simulink model "OvercurrentProtection"  (R2024a)
settings: Solver=ode23t  StartTime=0.0  StopTime=simulation.simTime  MaxStep=simulation.maxStepSize  RelTol=1e-3  AbsTol=1e-3
PostLoadFcn:
  | run('OvercurrentProtectionInput.mlx');
  | run('OvercurrentProtectionEstimateSettings.m');
InitFcn:
  | run('OvercurrentProtectionEstimateSettings.m');
undefined symbols (not defined in the file): distributionLine1, distributionLine2, fault, load, protection, relay1, relay2, source
libraries: ee_lib x27, fl_lib x17, eeGeneralControl x8, nesl_utility x7, simulink x4, simulink_extras x4
(part 1 of 2)
CloseFcn:
  | try, close(h1_OvercurrentProtectionPhase), end
  | clear h1_OvercurrentProtectionPhase
  | try, close(h2_OvercurrentProtectionEarth), end
  | clear h2_OvercurrentProtectionEarth
  | clear source;
  | clear transformer;
  | clear distributionLine1;
  | clear distributionLine2;
  | clear load;
  | clear sensor1;
  | clear sensor2;
  | clear fault;
  | clear protection;
  | clear maskParameter;
  | clear simlog_OvercurrentProtection;
  | clear simulation;
  | clear relay1;
  | clear relay2;
  | clear plotVar;
  | clear relayType;
  | clear mask;
Description:
  | Overcurrent Relay Protection in AC Microgrid
settings Model: Creator=The MathWorks, Inc.  LastModifiedBy=The MathWorks, Inc.
settings SolverCC: MaxConsecutiveZCs=100000  MaxConsecutiveMinStep=1000  MaxZcPerStep=1
settings DataIOCC: SaveOutput=off  SignalLogging=off  DSMLogging=off  SaveTime=off  ReturnWorkspaceOutputs=off
settings OptimizationCC: ReuseModelBlockBuffer=off
settings DebuggingCC: UnconnectedInputMsg=warning  UnconnectedOutputMsg=warning  UnconnectedLineMsg=warning
settings ModelReferenceCC: EnableRefExpFcnMdlSchedulingChecks=on
settings RTWCC: GPUComputeCapability=3.5  DLArmComputeVersion=19.05
settings SimscapeCC: SimscapeLogType=all  SimscapeLogName=simlog_OvercurrentProtection  SimscapeLogLimitData=off

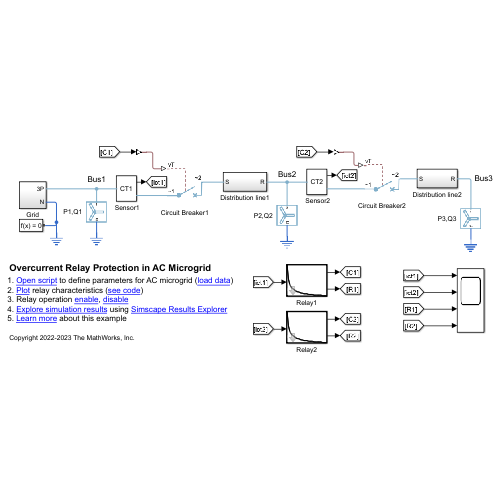
[thumbnail: Simulink's stored preview of the top-level diagram]
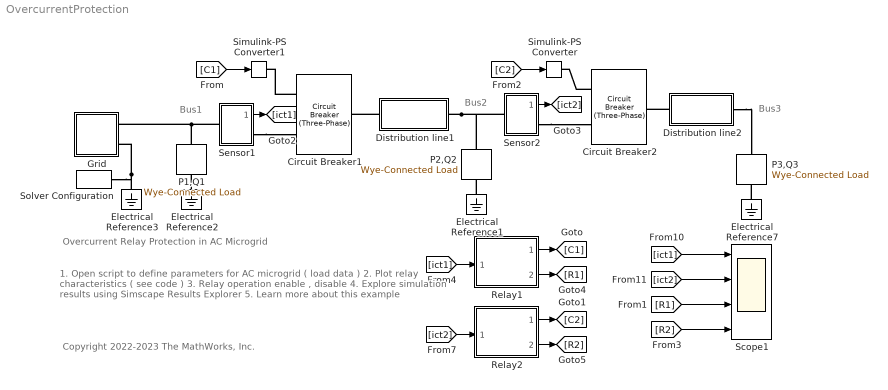
== system OvercurrentProtection ==
  note: Bus1
  note: Bus2
  note: Bus3
  note: Copyright 2022-2023 The MathWorks, Inc.
  note: Overcurrent Relay Protection in AC Microgrid
  note: 1. Open script to define parameters for AC microgrid ( load data )
      | 2. Plot relay characteristics ( see code )
      | 3. Relay operation enable , disable
      | 4. Explore simulation results using Simscape Results Explorer
      | 5. Learn more about this example
  " P2,Q2" : ee_lib/Passive/RLC Assemblies/Wye-Connected Load  parameterization=ee.enum.rlc.parameterization.ratedpower  component_structure=ee.enum.rlc.structure.R  component_structure_PQ=ee.enum.rlc.structure.SeriesRL  R=1 Ohm  L=1e-3 H  C=1e-6 F  VRated=transformer.secVoltage V  FRated=source.ratedFrequency Hz  P=load.P2 W  Qpos=load.Q2 V*A  Qneg=-1e2 V*A  R_parasitic=1e-6 Ohm  G_parasitic=1e-6 1/Ohm  R_parasitic_PQ=1e-6 Ohm  G_parasitic_PQ=1e-6 1/Ohm  Vmag0=33 kV  Vang0=0 deg  Freq0=50 Hz  IL_specify=off  IL_priority=High  IL=[ 0 0 0 ] A  IL_nominal_specify=off  IL_nominal_value=1  IL_nominal_unit=A  VC_specify=off  VC_priority=High  VC=[ 0 0 0 ] V  VC_nominal_specify=off  VC_nominal_value=1  VC_nominal_unit=V
  " Sensor1" : Subsystem
      mask Display: disp('CT1')
  " Sensor2" : Subsystem
      mask Display: disp('CT2')
  Circuit Breaker1 : ee_lib/Switches & Breakers/Circuit Breaker (Three-Phase)  R_closed=0.001 Ohm  G_open=1e-6 1/Ohm  threshold=0.5 V  breaker_behavior=ee.enum.switches.breakerBehavior.zeroCrossingEnable
      settings: InternalSimscapePortConfiguration="{\"Bottom\":[],\"Left\":[{\"id\":\"vT\",\"label\":\"vT\",\"type\":\"input\"},{\"id\":\"N1\",\"label\":\"~1\",\"type\":\"foundation.electrical.three_phase\"}],\"Right\":[{\"id\":\"N2\",\"label\":\"~2\",\"type\":\"foundation.electrical.three_phase\"}],\"Top\":[]}"
  Circuit Breaker2 : ee_lib/Switches & Breakers/Circuit Breaker (Three-Phase)  R_closed=0.001 Ohm  G_open=1e-6 1/Ohm  threshold=0.5 V  breaker_behavior=ee.enum.switches.breakerBehavior.zeroCrossingEnable
      settings: InternalSimscapePortConfiguration="{\"Bottom\":[],\"Left\":[{\"id\":\"vT\",\"label\":\"vT\",\"type\":\"input\"},{\"id\":\"N1\",\"label\":\"~1\",\"type\":\"foundation.electrical.three_phase\"}],\"Right\":[{\"id\":\"N2\",\"label\":\"~2\",\"type\":\"foundation.electrical.three_phase\"}],\"Top\":[]}"
  Distribution line1 : Subsystem
  Distribution line2 : Subsystem
  Electrical Reference{1..3,7} (4 alike) : fl_lib/Electrical/Electrical Elements/Electrical Reference
  Grid : Subsystem
  P1,Q1 : ee_lib/Passive/RLC Assemblies/Wye-Connected Load  parameterization=ee.enum.rlc.parameterization.ratedpower  component_structure=ee.enum.rlc.structure.R  component_structure_PQ=ee.enum.rlc.structure.SeriesRL  R=1 Ohm  L=1e-3 H  C=1e-6 F  VRated=transformer.secVoltage V  FRated=source.ratedFrequency Hz  P=load.P1 W  Qpos=load.Q1 V*A  Qneg=-1e2 V*A  R_parasitic=1e-6 Ohm  G_parasitic=1e-6 1/Ohm  R_parasitic_PQ=1e-6 Ohm  G_parasitic_PQ=1e-6 1/Ohm  Vmag0=33 kV  Vang0=0 deg  Freq0=50 Hz  IL_specify=off  IL_priority=High  IL=[ 0 0 0 ] A  IL_nominal_specify=off  IL_nominal_value=1  IL_nominal_unit=A  VC_specify=off  VC_priority=High  VC=[ 0 0 0 ] V  VC_nominal_specify=off  VC_nominal_value=1  VC_nominal_unit=V
  P3,Q3 : ee_lib/Passive/RLC Assemblies/Wye-Connected Load  parameterization=ee.enum.rlc.parameterization.ratedpower  component_structure=ee.enum.rlc.structure.R  component_structure_PQ=ee.enum.rlc.structure.SeriesRL  R=1 Ohm  L=1e-3 H  C=1e-6 F  VRated=transformer.secVoltage V  FRated=source.ratedFrequency Hz  P=load.P3 W  Qpos=load.Q3 V*A  Qneg=-1e2 V*A  R_parasitic=1e-6 Ohm  G_parasitic=1e-6 1/Ohm  R_parasitic_PQ=1e-6 Ohm  G_parasitic_PQ=1e-6 1/Ohm  Vmag0=33 kV  Vang0=0 deg  Freq0=50 Hz  IL_specify=off  IL_priority=High  IL=[ 0 0 0 ] A  IL_nominal_specify=off  IL_nominal_value=1  IL_nominal_unit=A  VC_specify=off  VC_priority=High  VC=[ 0 0 0 ] V  VC_nominal_specify=off  VC_nominal_value=1  VC_nominal_unit=V
  Relay1 : Subsystem  TreatAsAtomicUnit=on  SystemSampleTime=relay1.sampleTime  mask{relayCharacteristicPhase=IEEE Moderately Inverse, relayCharacteristicEarth=IEEE Moderately Inverse, ratedFrequency=source.ratedFrequency, sampleTime=relay1.sampleTime, protectionEnable=protection.enable, currentPhase=[1.5 2.5 3.5 4.5 5.5 6.5 7.5 8.5 9.5 10.5], tmsPhase=[0.1 0.2], topPhase=[0.64 1.29;0.29 0.58;0.21 0.43;0.18 0.36;0.16 0.32;0.15 0.29;0.14 0.27;0.13 0.26;0.12 0.25;0.12 0.24], currentEarth=[0.06 0.15 0.2 0.25 0.3 0.35 0.4 0.45 0.5 0.55], tmsEarth=[0.1 0.2], topEarth=[0.64 1.29;0.29 0.58;0.21 0.43;0.18 0.36;0.16 0.32;0.15 0.29;0.14 0.27;0.13 0.26;0.12 0.25;0.12 0.24], phPickUp=relay1.phFltPickUp, ethPickUp=relay1.erFltPickUp, phTimeSetting=relay1.phFltTMS, ethTimeSetting=relay1.erFltTMS, topPhaseActual=0.2, topEarthActual=0.3}
      mask prompts: relayCharacteristicPhase "Relay characteristics for phase protection"; relayCharacteristicEarth "Relay characteristics for earth protection"; ratedFrequency "Fundamental frequency (Hz)"; sampleTime "Relay sample time (s)"; protectionEnable "Relay operation enable"; currentPhase "Current setting for phase protection (A)"; tmsPhase "Time multiplier setting for phase protection (s)"; topPhase "Operating time for phase protection (s)"; currentEarth "Current setting for earth protection (A)"; tmsEarth "Time multiplier setting for earth protection (s)"; topEarth "Operating time for earth protection (s)"; phPickUp "Pick up current for phase protection (A)"; ethPickUp "Pick up current for earth protection (A)"; phTimeSetting "Time multiplier setting for phase protection (s)"; ethTimeSetting "Time multiplier setting for earth protection (s)"; topPhaseActual "Relay operating time for phase protection (s)"; topEarthActual "Relay operating time for earth protection (s)"
      mask TypeOptions relayCharacteristicPhase: IEC Normal Inverse | IEC Very Inverse | IEC Extremely Inverse | IEEE Moderately Inverse | IEEE Very Inverse | IEEE Extremely Inverse | Definite Time | IvsT
      mask Callback relayCharacteristicPhase:
      | % Control parameter visiblity
      | enablePhase = get_param(gcb,'relayCharacteristicPhase');
      | enableEarth = get_param(gcb,'relayCharacteristicEarth');
      | % Set the 'MaskVisibilities' property for each parameters
      | cArray=cell(1,17);
      | cArray(:)={'on'};
      | p=strcmp(enablePhase,'IvsT');
      | q=strcmp(enableEarth,'IvsT');
      | r=strcmp(enablePhase,'Definite Time');
      | s=strcmp(enableEarth,'Definite Time');
      | if p==0 && q==1
      |     cArray(6:8)={'off'};
      | elseif p==0 && q==0
      |     cArray(6:11)={'off'};
      | elseif p==1 && q==0
      |     cArray(9:11)={'off'};
      | end
      | if r==0 && s==1
      |     cArray(15)={'off'};
      |     cArray(16)={'off'};
      | elseif r==0 && s==0
      |     cArray(16:17)={'off'};
      | elseif r==1 && s==0
      |     cArray(14)={'off'};
      |     cArray(17)={'off'};
      | elseif r==1 && s==1
      |     cArray(14:15)={'off'};
      | end
      | set_param(gcb,'MaskVisibilities',cArray);
      mask TypeOptions relayCharacteristicEarth: IEC Normal Inverse | IEC Very Inverse | IEC Extremely Inverse | IEEE Moderately Inverse | IEEE Very Inverse | IEEE Extremely Inverse | Definite Time | IvsT
      mask Callback relayCharacteristicEarth:
      | % Control parameter visiblity
      | enablePhase = get_param(gcb,'relayCharacteristicPhase');
      | enableEarth = get_param(gcb,'relayCharacteristicEarth');
      | % Set the 'MaskVisibilities' property for each parameters
      | cArray=cell(1,17);
      | cArray(:)={'on'};
      | p=strcmp(enablePhase,'IvsT');
      | q=strcmp(enableEarth,'IvsT');
      | r=strcmp(enablePhase,'Definite Time');
      | s=strcmp(enableEarth,'Definite Time');
      | if p==0 && q==1
      |     cArray(6:8)={'off'};
      | elseif p==0 && q==0
      |     cArray(6:11)={'off'};
      | elseif p==1 && q==0
      |     cArray(9:11)={'off'};
      | end
      | if r==0 && s==1
      |     cArray(15)={'off'};
      |     cArray(16)={'off'};
      | elseif r==0 && s==0
      |     cArray(16:17)={'off'};
      | elseif r==1 && s==0
      |     cArray(14)={'off'};
      |     cArray(17)={'off'};
      | elseif r==1 && s==1
      |     cArray(14:15)={'off'};
      | end
      | set_param(gcb,'MaskVisibilities',cArray);
      mask DialogControl Container9 Prompt: Main
      mask DialogControl Container24 Prompt: Current Settings
      mask DialogControl Container19 Prompt: Time Settings
      mask Display:
      | psm = 1:1:30; % Plug setting multiplier
      | tms=0.01; % Time multiplier setting is assumed to be 0.01s
      | top=ones(2,length(psm));  % Operating time of the relay
      | maskParameter=Simulink.Mask.get(gcb); % Get the mask parameters
      | for i=1:2
      |     index(i)=find(strcmp(maskParameter.Parameters(1,i).Value,maskParameter.Parameters(1,i).TypeOptions));
      |     if index(i)<7
      |         switch index(i)              % Selection of relay characteristic
      |             case 1                   % IEC Normal Inverse
      |                 a=0.14;
      |                 b=0.02;
      |                 c=0;
      |             case 2                   % IEC Very Inverse
      |                 a=13.5;
      |                 b=1;
      |                 c=0;
      |             case 3                   % IEC Extremely Inverse
      |                 a=80;
      |                 b=2;
      |                 c=0;
      |             case 4                   % IEEE Moderately Inverse
      |                 a=0.0515;
      |                 b=0.02;
      |                 c=0.114;
      |             case 5                   % IEEE Very Inverse
      |                 a=19.61;
      |                 b=2;
      |                 c=0.491;
      |             otherwise                % IEEE Exteremely Inverse
      |                 a=28.2;
      |                 b=2;
      |                 c=0.1217;
      |         end
      |         for j=1:length(psm)
      |             top(i,j)=tms*((a/(power(psm(j),b)-1))+c); % Operating time of the relay
      |         end
      |     else
      |         top(i,1:length(psm))=0.03*ones(1,length(psm));% Operating time of the relay
      |     end
      | end
      | top1=top(1,1:end);
      | top2=top(2,1:end);
      | 
      | maskFigure=figure;
      | if index(1)<8
      |     plot(psm,top1)
      | else
      |     fprintf('\n\nIvsT');
      | end
      | hold on;
      | if index(2)<8
      |     plot(psm,top2);
      | elseif index(1)<8
      |     fprintf('\nIvsT');
      | end
      | close(maskFigure);
  Relay2 : Subsystem  TreatAsAtomicUnit=on  SystemSampleTime=relay1.sampleTime  mask{relayCharacteristicPhase=IEEE Moderately Inverse, relayCharacteristicEarth=IEEE Moderately Inverse, ratedFrequency=source.ratedFrequency, sampleTime=relay2.sampleTime, protectionEnable=protection.enable, currentPhase=[1.5 2.5 3.5 4.5 5.5 6.5 7.5 8.5 9.5 10.5], tmsPhase=[0.1 0.2], topPhase=[0.64 1.29;0.29 0.58;0.21 0.43;0.18 0.36;0.16 0.32;0.15 0.29;0.14 0.27;0.13 0.26;0.12 0.25;0.12 0.24], currentEarth=[0.06 0.15 0.2 0.25 0.3 0.35 0.4 0.45 0.5 0.55], tmsEarth=[0.1 0.2], topEarth=[0.64 1.29;0.29 0.58;0.21 0.43;0.18 0.36;0.16 0.32;0.15 0.29;0.14 0.27;0.13 0.26;0.12 0.25;0.12 0.24], phPickUp=relay2.phFltPickUp, ethPickUp=relay2.erFltPickUp, phTimeSetting=relay2.phFltTMS, ethTimeSetting=relay2.erFltTMS, topPhaseActual=0.2, topEarthActual=0.3}
      mask prompts: relayCharacteristicPhase "Relay characteristics for phase protection"; relayCharacteristicEarth "Relay characteristics for earth protection"; ratedFrequency "Fundamental frequency (Hz)"; sampleTime "Relay sample time (s)"; protectionEnable "Relay operation enable"; currentPhase "Current setting for phase protection (A)"; tmsPhase "Time multiplier setting for phase protection (s)"; topPhase "Operating time for phase protection (s)"; currentEarth "Current setting for earth protection (A)"; tmsEarth "Time multiplier setting for earth protection (s)"; topEarth "Operating time for earth protection (s)"; phPickUp "Pick up current for phase protection (A)"; ethPickUp "Pick up current for earth protection (A)"; phTimeSetting "Time multiplier setting for phase protection (s)"; ethTimeSetting "Time multiplier setting for earth protection (s)"; topPhaseActual "Relay operating time for phase protection (s)"; topEarthActual "Relay operating time for earth protection (s)"
      mask TypeOptions relayCharacteristicPhase: IEC Normal Inverse | IEC Very Inverse | IEC Extremely Inverse | IEEE Moderately Inverse | IEEE Very Inverse | IEEE Extremely Inverse | Definite Time | IvsT
      mask Callback relayCharacteristicPhase:
      | % Control parameter visiblity
      | enablePhase = get_param(gcb,'relayCharacteristicPhase');
      | enableEarth = get_param(gcb,'relayCharacteristicEarth');
      | % Set the 'MaskVisibilities' property for each parameters
      | cArray=cell(1,17);
      | cArray(:)={'on'};
      | p=strcmp(enablePhase,'IvsT');
      | q=strcmp(enableEarth,'IvsT');
      | r=strcmp(enablePhase,'Definite Time');
      | s=strcmp(enableEarth,'Definite Time');
      | if p==0 && q==1
      |     cArray(6:8)={'off'};
      | elseif p==0 && q==0
      |     cArray(6:11)={'off'};
      | elseif p==1 && q==0
      |     cArray(9:11)={'off'};
      | end
      | if r==0 && s==1
      |     cArray(15)={'off'};
      |     cArray(16)={'off'};
      | elseif r==0 && s==0
      |     cArray(16:17)={'off'};
      | elseif r==1 && s==0
      |     cArray(14)={'off'};
      |     cArray(17)={'off'};
      | elseif r==1 && s==1
      |     cArray(14:15)={'off'};
      | end
      | set_param(gcb,'MaskVisibilities',cArray);
      mask TypeOptions relayCharacteristicEarth: IEC Normal Inverse | IEC Very Inverse | IEC Extremely Inverse | IEEE Moderately Inverse | IEEE Very Inverse | IEEE Extremely Inverse | Definite Time | IvsT
      mask Callback relayCharacteristicEarth:
      | % Control parameter visiblity
      | enablePhase = get_param(gcb,'relayCharacteristicPhase');
      | enableEarth = get_param(gcb,'relayCharacteristicEarth');
      | % Set the 'MaskVisibilities' property for each parameters
      | cArray=cell(1,17);
      | cArray(:)={'on'};
      | p=strcmp(enablePhase,'IvsT');
      | q=strcmp(enableEarth,'IvsT');
      | r=strcmp(enablePhase,'Definite Time');
      | s=strcmp(enableEarth,'Definite Time');
      | if p==0 && q==1
      |     cArray(6:8)={'off'};
      | elseif p==0 && q==0
      |     cArray(6:11)={'off'};
      | elseif p==1 && q==0
      |     cArray(9:11)={'off'};
      | end
      | if r==0 && s==1
      |     cArray(15)={'off'};
      |     cArray(16)={'off'};
      | elseif r==0 && s==0
      |     cArray(16:17)={'off'};
      | elseif r==1 && s==0
      |     cArray(14)={'off'};
      |     cArray(17)={'off'};
      | elseif r==1 && s==1
      |     cArray(14:15)={'off'};
      | end
      | set_param(gcb,'MaskVisibilities',cArray);
      mask DialogControl Container9 Prompt: Main
      mask DialogControl Container24 Prompt: Current Settings
      mask DialogControl Container19 Prompt: Time Settings
      mask Display:
      | psm = 1:1:30; % Plug setting multiplier
      | tms=0.01; % Time multiplier setting is assumed to be 0.01s
      | top=ones(2,length(psm));  % Operating time of the relay
      | maskParameter=Simulink.Mask.get(gcb); % Get the mask parameters
      | for i=1:2
      |     index(i)=find(strcmp(maskParameter.Parameters(1,i).Value,maskParameter.Parameters(1,i).TypeOptions));
      |     if index(i)<7
      |         switch index(i)              % Selection of relay characteristic
      |             case 1                   % IEC Normal Inverse
      |                 a=0.14;
      |                 b=0.02;
      |                 c=0;
      |             case 2                   % IEC Very Inverse
      |                 a=13.5;
      |                 b=1;
      |                 c=0;
      |             case 3                   % IEC Extremely Inverse
      |                 a=80;
      |                 b=2;
      |                 c=0;
      |             case 4                   % IEEE Moderately Inverse
      |                 a=0.0515;
      |                 b=0.02;
      |                 c=0.114;
      |             case 5                   % IEEE Very Inverse
      |                 a=19.61;
      |                 b=2;
      |                 c=0.491;
      |             otherwise                % IEEE Exteremely Inverse
      |                 a=28.2;
      |                 b=2;
      |                 c=0.1217;
      |         end
      |         for j=1:length(psm)
      |             top(i,j)=tms*((a/(power(psm(j),b)-1))+c); % Operating time of the relay
      |         end
      |     else
      |         top(i,1:length(psm))=0.03*ones(1,length(psm));% Operating time of the relay
      |     end
      | end
      | top1=top(1,1:end);
      | top2=top(2,1:end);
      | 
      | maskFigure=figure;
      | if index(1)<8
      |     plot(psm,top1)
      | else
      |     fprintf('\n\nIvsT');
      | end
      | hold on;
      | if index(2)<8
      |     plot(psm,top2);
      | elseif index(1)<8
      |     fprintf('\nIvsT');
      | end
      | close(maskFigure);
  Scope1 : Scope  NumInputPorts=4
  Simulink-PS Converter : nesl_utility/Simulink-PS Converter  PhysicalDomain=network_engine_domain  SubClassName=ps_input  LeftPortType=input  RightPortType=output  PseudoPeriodic=off  Frequencies=[]  NoiseDistribution=none  NoiseParameters=[]  Unit=1  AffineConversion=off  FilteringAndDerivatives=zero  SimscapeFilterOrder=1  InputFilterTimeConstant=0.001  UdotUserProvided=0
  Simulink-PS Converter1 : nesl_utility/Simulink-PS Converter  PhysicalDomain=network_engine_domain  SubClassName=ps_input  LeftPortType=input  RightPortType=output  PseudoPeriodic=off  Frequencies=[]  NoiseDistribution=none  NoiseParameters=[]  Unit=1  AffineConversion=off  FilteringAndDerivatives=zero  SimscapeFilterOrder=1  InputFilterTimeConstant=0.001  UdotUserProvided=0
  Solver Configuration : nesl_utility/Solver Configuration  PhysicalDomain=network_engine_domain  SubClassName=solver  LeftPortType=input  RightPortType=generic  Tones=[]  Harmonics=[]  SimulateNoise=off  Profile=off  UseLocalSampling=off  EnableSwitchedLinearOptims=on  FrequencyDomain=off  UseCCode=off  RelTol=0.001  AbsTol=1e-06  MinStep=1e-09  ToWorkspace=off  RevertToSquareIcSolve=off  NumHomotopyIterations=100  PhasorMode=off  PhasorModeNumHarmonics=1  ConsistencySolver=NEWTON_FTOL  IndexReductionMethod=DerivativeReplacement  DoDC=on  ResidualTolerance=1e-9  ConsistencyTolSource=GLOBAL  ConsistencyAbsTol=0.001  ConsistencyRelTol=0.001  ConsistencyTolFactor=0.001  UseLocalSolver=off  LocalSolverChoice=NE_BACKWARD_EULER_ADVANCER  ResolveIndetEquations=on  FunctionEvalNumThread=1  LocalSolverSampleTime=1e-4  DoFixedCost=off  MaxNonlinIter=10  MaxModeIter=2  ComputeImpulses=off  ImpulseIterations=2  LinearAlgebra=auto  LinearAlgebraNumThread=0  EquationFormulation=NE_TIME_EF  DelaysMemoryBudget=4096  AutomaticFiltering=off  FilteringTimeConstant=0.0001  PartitionStorageMethod=AS_NEEDED  PartitionMemoryBudget=1024  PartitionMethod=FAST  MultibodyUseLocalSolver=off  MultibodyLocalSolverChoice=ODE1  MultibodyLocalSolverSampleTime=0.001
  wires:
  Relay1/1(Trip Signal) -> [C1]
  " Sensor1"/1(Out1) -> [ict1]
  [ict1] -> Relay1/1(Inport)
  Relay2/1(Trip Signal) -> [C2]
  [C2] -> Simulink-PS Converter/1
  [R2] -> Scope1/4
  [C1] -> Simulink-PS Converter1/1
  [R1] -> Scope1/3
  " Sensor2"/1(Out1) -> [ict2]
  Relay1/2(Relay Status) -> [R1]
  [ict2] -> Relay2/1(Inport)
  Relay2/2(Relay Status) -> [R2]
  [ict1] -> Scope1/1
  [ict2] -> Scope1/2
  connections:
  Solver Configuration/RConn1 -- Electrical Reference3/LConn1 -- Grid/RConn2
  P1,Q1/LConn1 -- " Sensor1"/LConn1 -- Grid/RConn1
  Distribution line1/RConn1 -- " Sensor2"/LConn1 -- " P2,Q2"/LConn1
  Circuit Breaker2/LConn1 -- Simulink-PS Converter/RConn1
  " Sensor1"/RConn1 -- Circuit Breaker1/LConn2
  Electrical Reference1/LConn1 -- " P2,Q2"/RConn1
  Distribution line2/RConn1 -- P3,Q3/LConn1
  Circuit Breaker1/LConn1 -- Simulink-PS Converter1/RConn1
  Distribution line2/LConn1 -- Circuit Breaker2/RConn1
  Distribution line1/LConn1 -- Circuit Breaker1/RConn1
  Electrical Reference7/LConn1 -- P3,Q3/RConn1
  " Sensor2"/RConn1 -- Circuit Breaker2/LConn2
  Electrical Reference2/LConn1 -- P1,Q1/RConn1

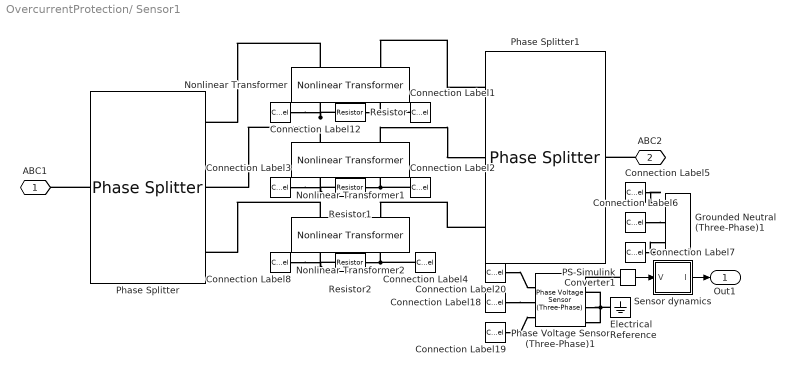
== system OvercurrentProtection/ Sensor1 ==
  Connection Label1 : ConnectionLabel  Label=Ian
  Connection Label12 : ConnectionLabel  Label=Iap
  Connection Label18 : ConnectionLabel  Label=Ibp
  Connection Label19 : ConnectionLabel  Label=Icp
  Connection Label2 : ConnectionLabel  Label=Ibn
  Connection Label20 : ConnectionLabel  Label=Iap
  Connection Label3 : ConnectionLabel  Label=Ibp
  Connection Label4 : ConnectionLabel  Label=Ibn
  Connection Label5 : ConnectionLabel  Label=Ian
  Connection Label6 : ConnectionLabel  Label=Ibn
  Connection Label7 : ConnectionLabel  Label=Icn
  Connection Label8 : ConnectionLabel  Label=Icp
  Electrical Reference : fl_lib/Electrical/Electrical Elements/Electrical Reference
  Grounded Neutral (Three-Phase)1 : ee_lib/Connectors & References/Grounded Neutral (Three-Phase)
      settings: InternalSimscapePortConfiguration="{\"Bottom\":[],\"Left\":[{\"id\":\"a\",\"label\":\"a\",\"type\":\"foundation.electrical.electrical\"},{\"id\":\"b\",\"label\":\"b\",\"type\":\"foundation.electrical.electrical\"},{\"id\":\"c\",\"label\":\"c\",\"type\":\"foundation.electrical.electrical\"}],\"Right\":[],\"Top\":[]}"
  Nonlinear Transformer : ee_lib/Passive/Transformers/Nonlinear Transformer  Nw=1  Nw2=sensor1.ctRatio  winding_param_option=1  Req=1e-3 Ohm  Leq=1e-4 H  R_1=0.01 Ohm  L_1=0.0001 H  R_2=0.01 Ohm  L_2=0.0001 H  averaging_period=0 s  R_m=100 Ohm  parameterization_option=1  H_data=[0, 200, 400, 600, 800, 1000] A/m  B_data=[0, .81, 1.25, 1.42, 1.48, 1.49] T  length_effective=0.2 m  area_effective=2e-4 m^2  L=4e-2 H  L_sat=1e-2 H  current_data=[0, .4, .8, 1.2, 1.6, 2] A  magnetic_flux_data=[0, .161, .25, .284, .295, .299] .* 1e-3 Wb  magnetic_flux_sat=1.6e-04 Wb  dBdH0=0.005 m*T/A  B1=1.49 T  H1=1000 A/m  c=0.1  K=200 A/m  alpha=1e-4  interpolation_option=1  Leq_i0=0 A  L1_i0=0 A  L2_i0=0 A  x0_option=1  i_L0=0 A  phi0=0 Wb  B0=0 T  H0=0 A/m  Leq_g=1e-9 1/Ohm  L1_g=1e-9 1/Ohm  L2_g=1e-9 1/Ohm
      settings: InternalSimscapePortConfiguration="{\"Bottom\":[],\"Left\":[{\"id\":\"p1\",\"label\":\"1+\",\"type\":\"foundation.electrical.electrical\"},{\"id\":\"n1\",\"label\":\"1-\",\"type\":\"foundation.electrical.electrical\"}],\"Right\":[{\"id\":\"p2\",\"label\":\"2+\",\"type\":\"foundation.electrical.electrical\"},{\"id\":\"n2\",\"label\":\"2-\",\"type\":\"foundation.electrical.electrical\"}],\"Top\":[]}"
  Nonlinear Transformer1 : ee_lib/Passive/Transformers/Nonlinear Transformer  Nw=1  Nw2=sensor1.ctRatio  winding_param_option=1  Req=1e-3 Ohm  Leq=1e-4 H  R_1=0.01 Ohm  L_1=0.0001 H  R_2=0.01 Ohm  L_2=0.0001 H  averaging_period=0 s  R_m=100 Ohm  parameterization_option=1  H_data=[0, 200, 400, 600, 800, 1000] A/m  B_data=[0, .81, 1.25, 1.42, 1.48, 1.49] T  length_effective=0.2 m  area_effective=2e-4 m^2  L=4e-2 H  L_sat=1e-2 H  current_data=[0, .4, .8, 1.2, 1.6, 2] A  magnetic_flux_data=[0, .161, .25, .284, .295, .299] .* 1e-3 Wb  magnetic_flux_sat=1.6e-04 Wb  dBdH0=0.005 m*T/A  B1=1.49 T  H1=1000 A/m  c=0.1  K=200 A/m  alpha=1e-4  interpolation_option=1  Leq_i0=0 A  L1_i0=0 A  L2_i0=0 A  x0_option=1  i_L0=0 A  phi0=0 Wb  B0=0 T  H0=0 A/m  Leq_g=1e-9 1/Ohm  L1_g=1e-9 1/Ohm  L2_g=1e-9 1/Ohm
      settings: InternalSimscapePortConfiguration="{\"Bottom\":[],\"Left\":[{\"id\":\"p1\",\"label\":\"1+\",\"type\":\"foundation.electrical.electrical\"},{\"id\":\"n1\",\"label\":\"1-\",\"type\":\"foundation.electrical.electrical\"}],\"Right\":[{\"id\":\"p2\",\"label\":\"2+\",\"type\":\"foundation.electrical.electrical\"},{\"id\":\"n2\",\"label\":\"2-\",\"type\":\"foundation.electrical.electrical\"}],\"Top\":[]}"
  Nonlinear Transformer2 : ee_lib/Passive/Transformers/Nonlinear Transformer  Nw=1  Nw2=sensor1.ctRatio  winding_param_option=1  Req=1e-3 Ohm  Leq=1e-4 H  R_1=0.01 Ohm  L_1=0.0001 H  R_2=0.01 Ohm  L_2=0.0001 H  averaging_period=0 s  R_m=100 Ohm  parameterization_option=1  H_data=[0, 200, 400, 600, 800, 1000] A/m  B_data=[0, .81, 1.25, 1.42, 1.48, 1.49] T  length_effective=0.2 m  area_effective=2e-4 m^2  L=4e-2 H  L_sat=1e-2 H  current_data=[0, .4, .8, 1.2, 1.6, 2] A  magnetic_flux_data=[0, .161, .25, .284, .295, .299] .* 1e-3 Wb  magnetic_flux_sat=1.6e-04 Wb  dBdH0=0.005 m*T/A  B1=1.49 T  H1=1000 A/m  c=0.1  K=200 A/m  alpha=1e-4  interpolation_option=1  Leq_i0=0 A  L1_i0=0 A  L2_i0=0 A  x0_option=1  i_L0=0 A  phi0=0 Wb  B0=0 T  H0=0 A/m  Leq_g=1e-9 1/Ohm  L1_g=1e-9 1/Ohm  L2_g=1e-9 1/Ohm
      settings: InternalSimscapePortConfiguration="{\"Bottom\":[],\"Left\":[{\"id\":\"p1\",\"label\":\"1+\",\"type\":\"foundation.electrical.electrical\"},{\"id\":\"n1\",\"label\":\"1-\",\"type\":\"foundation.electrical.electrical\"}],\"Right\":[{\"id\":\"p2\",\"label\":\"2+\",\"type\":\"foundation.electrical.electrical\"},{\"id\":\"n2\",\"label\":\"2-\",\"type\":\"foundation.electrical.electrical\"}],\"Top\":[]}"
  PS-Simulink Converter1 : nesl_utility/PS-Simulink Converter  PhysicalDomain=network_engine_domain  SubClassName=ps_output  LeftPortType=input  RightPortType=output  PseudoPeriodic=off  Frequencies=[]  VectorFormat=1-D array  Unit=inherit  AffineConversion=off
  Phase Splitter : ee_lib/Connectors & References/Phase Splitter
  Phase Splitter1 : ee_lib/Connectors & References/Phase Splitter
  Phase Voltage Sensor (Three-Phase)1 : ee_lib/Sensors & Transducers/Phase Voltage Sensor (Three-Phase)
      settings: LogSimulationData=on  InternalSimscapePortConfiguration="{\"Bottom\":[],\"Left\":[{\"id\":\"a1\",\"label\":\"a1\",\"type\":\"foundation.electrical.electrical\"},{\"id\":\"b1\",\"label\":\"b1\",\"type\":\"foundation.electrical.electrical\"},{\"id\":\"c1\",\"label\":\"c1\",\"type\":\"foundation.electrical.electrical\"}],\"Right\":[{\"id\":\"V_output\",\"label\":\"V\",\"type\":\"output\"},{\"id\":\"a2\",\"label\":\"a2\",\"type\":\"foundation.electrical.electrical\"},{\"id\":\"b2\",\"label\":\"b2\",\"type\":\"foundation.electrical.electrical\"},{\"id\":\"c2\",\"label\":\"c2\",\"type\":\"foundation.electrical.electrical\"}],\"Top\":[]}"
  Resistor : fl_lib/Electrical/Electrical Elements/Resistor  R=1 Ohm  i_specify=off  i_priority=None  i=0 A  i_nominal_specify=off  i_nominal_value=1  i_nominal_unit=A  v_specify=off  v_priority=None  v=0 V  v_nominal_specify=off  v_nominal_value=1  v_nominal_unit=V
  Resistor1 : fl_lib/Electrical/Electrical Elements/Resistor  R=1 Ohm  i_specify=off  i_priority=None  i=0 A  i_nominal_specify=off  i_nominal_value=1  i_nominal_unit=A  v_specify=off  v_priority=None  v=0 V  v_nominal_specify=off  v_nominal_value=1  v_nominal_unit=V
  Resistor2 : fl_lib/Electrical/Electrical Elements/Resistor  R=1 Ohm  i_specify=off  i_priority=None  i=0 A  i_nominal_specify=off  i_nominal_value=1  i_nominal_unit=A  v_specify=off  v_priority=None  v=0 V  v_nominal_specify=off  v_nominal_value=1  v_nominal_unit=V
  Sensor dynamics : Subsystem
  ABC1 : PMIOPort  Side=Left
  ABC2 : PMIOPort  Port=2  Side=Right
  Out1 : Outport
  wires:
  PS-Simulink Converter1/1 -> Sensor dynamics/1(V)
  Sensor dynamics/1(I) -> Out1/1
  connections:
  Phase Splitter/LConn1 -- ABC1/RConn1
  ABC2/RConn1 -- Phase Splitter1/LConn1
  Connection Label19/LConn1 -- Phase Voltage Sensor (Three-Phase)1/LConn3
  Connection Label18/LConn1 -- Phase Voltage Sensor (Three-Phase)1/LConn2
  PS-Simulink Converter1/LConn1 -- Phase Voltage Sensor (Three-Phase)1/RConn1
  Connection Label20/LConn1 -- Phase Voltage Sensor (Three-Phase)1/LConn1
  Nonlinear Transformer/RConn1 -- Resistor/LConn1 -- Connection Label12/LConn1
  Nonlinear Transformer/LConn1 -- Phase Splitter/RConn1
  Phase Splitter1/RConn1 -- Nonlinear Transformer/LConn2
  Resistor/RConn1 -- Connection Label1/LConn1 -- Nonlinear Transformer/RConn2
  Nonlinear Transformer1/RConn1 -- Resistor1/LConn1 -- Connection Label3/LConn1
  Nonlinear Transformer1/LConn2 -- Phase Splitter1/RConn2
  Nonlinear Transformer1/LConn1 -- Phase Splitter/RConn2
  Nonlinear Transformer2/RConn1 -- Resistor2/LConn1 -- Connection Label8/LConn1
  Nonlinear Transformer2/LConn1 -- Phase Splitter/RConn3
  Phase Splitter1/RConn3 -- Nonlinear Transformer2/LConn2
  Resistor2/RConn1 -- Connection Label4/LConn1 -- Nonlinear Transformer2/RConn2
  Resistor1/RConn1 -- Nonlinear Transformer1/RConn2 -- Connection Label2/LConn1
  Electrical Reference/LConn1 -- Phase Voltage Sensor (Three-Phase)1/RConn2 -- Phase Voltage Sensor (Three-Phase)1/RConn3 -- Phase Voltage Sensor (Three-Phase)1/RConn4
  Connection Label5/LConn1 -- Grounded Neutral (Three-Phase)1/LConn1
  Connection Label6/LConn1 -- Grounded Neutral (Three-Phase)1/LConn2
  Connection Label7/LConn1 -- Grounded Neutral (Three-Phase)1/LConn3

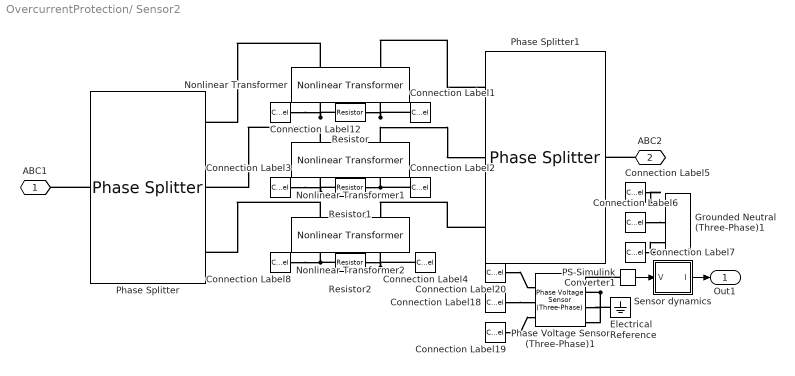
== system OvercurrentProtection/ Sensor2 ==
  Connection Label1 : ConnectionLabel  Label=Ian
  Connection Label12 : ConnectionLabel  Label=Iap
  Connection Label18 : ConnectionLabel  Label=Ibp
  Connection Label19 : ConnectionLabel  Label=Icp
  Connection Label2 : ConnectionLabel  Label=Ibn
  Connection Label20 : ConnectionLabel  Label=Iap
  Connection Label3 : ConnectionLabel  Label=Ibp
  Connection Label4 : ConnectionLabel  Label=Ibn
  Connection Label5 : ConnectionLabel  Label=Ian
  Connection Label6 : ConnectionLabel  Label=Ibn
  Connection Label7 : ConnectionLabel  Label=Icn
  Connection Label8 : ConnectionLabel  Label=Icp
  Electrical Reference : fl_lib/Electrical/Electrical Elements/Electrical Reference
  Grounded Neutral (Three-Phase)1 : ee_lib/Connectors & References/Grounded Neutral (Three-Phase)
      settings: InternalSimscapePortConfiguration="{\"Bottom\":[],\"Left\":[{\"id\":\"a\",\"label\":\"a\",\"type\":\"foundation.electrical.electrical\"},{\"id\":\"b\",\"label\":\"b\",\"type\":\"foundation.electrical.electrical\"},{\"id\":\"c\",\"label\":\"c\",\"type\":\"foundation.electrical.electrical\"}],\"Right\":[],\"Top\":[]}"
  Nonlinear Transformer : ee_lib/Passive/Transformers/Nonlinear Transformer  Nw=1  Nw2=sensor2.ctRatio  winding_param_option=1  Req=1e-3 Ohm  Leq=1e-4 H  R_1=0.01 Ohm  L_1=0.0001 H  R_2=0.01 Ohm  L_2=0.0001 H  averaging_period=0 s  R_m=100 Ohm  parameterization_option=1  H_data=[0, 200, 400, 600, 800, 1000] A/m  B_data=[0, .81, 1.25, 1.42, 1.48, 1.49] T  length_effective=0.2 m  area_effective=2e-4 m^2  L=4e-2 H  L_sat=1e-2 H  current_data=[0, .4, .8, 1.2, 1.6, 2] A  magnetic_flux_data=[0, .161, .25, .284, .295, .299] .* 1e-3 Wb  magnetic_flux_sat=1.6e-04 Wb  dBdH0=0.005 m*T/A  B1=1.49 T  H1=1000 A/m  c=0.1  K=200 A/m  alpha=1e-4  interpolation_option=1  Leq_i0=0 A  L1_i0=0 A  L2_i0=0 A  x0_option=1  i_L0=0 A  phi0=0 Wb  B0=0 T  H0=0 A/m  Leq_g=1e-9 1/Ohm  L1_g=1e-9 1/Ohm  L2_g=1e-9 1/Ohm
      settings: InternalSimscapePortConfiguration="{\"Bottom\":[],\"Left\":[{\"id\":\"p1\",\"label\":\"1+\",\"type\":\"foundation.electrical.electrical\"},{\"id\":\"n1\",\"label\":\"1-\",\"type\":\"foundation.electrical.electrical\"}],\"Right\":[{\"id\":\"p2\",\"label\":\"2+\",\"type\":\"foundation.electrical.electrical\"},{\"id\":\"n2\",\"label\":\"2-\",\"type\":\"foundation.electrical.electrical\"}],\"Top\":[]}"
  Nonlinear Transformer1 : ee_lib/Passive/Transformers/Nonlinear Transformer  Nw=1  Nw2=sensor2.ctRatio  winding_param_option=1  Req=1e-3 Ohm  Leq=1e-4 H  R_1=0.01 Ohm  L_1=0.0001 H  R_2=0.01 Ohm  L_2=0.0001 H  averaging_period=0 s  R_m=100 Ohm  parameterization_option=1  H_data=[0, 200, 400, 600, 800, 1000] A/m  B_data=[0, .81, 1.25, 1.42, 1.48, 1.49] T  length_effective=0.2 m  area_effective=2e-4 m^2  L=4e-2 H  L_sat=1e-2 H  current_data=[0, .4, .8, 1.2, 1.6, 2] A  magnetic_flux_data=[0, .161, .25, .284, .295, .299] .* 1e-3 Wb  magnetic_flux_sat=1.6e-04 Wb  dBdH0=0.005 m*T/A  B1=1.49 T  H1=1000 A/m  c=0.1  K=200 A/m  alpha=1e-4  interpolation_option=1  Leq_i0=0 A  L1_i0=0 A  L2_i0=0 A  x0_option=1  i_L0=0 A  phi0=0 Wb  B0=0 T  H0=0 A/m  Leq_g=1e-9 1/Ohm  L1_g=1e-9 1/Ohm  L2_g=1e-9 1/Ohm
      settings: InternalSimscapePortConfiguration="{\"Bottom\":[],\"Left\":[{\"id\":\"p1\",\"label\":\"1+\",\"type\":\"foundation.electrical.electrical\"},{\"id\":\"n1\",\"label\":\"1-\",\"type\":\"foundation.electrical.electrical\"}],\"Right\":[{\"id\":\"p2\",\"label\":\"2+\",\"type\":\"foundation.electrical.electrical\"},{\"id\":\"n2\",\"label\":\"2-\",\"type\":\"foundation.electrical.electrical\"}],\"Top\":[]}"
  Nonlinear Transformer2 : ee_lib/Passive/Transformers/Nonlinear Transformer  Nw=1  Nw2=sensor2.ctRatio  winding_param_option=1  Req=1e-3 Ohm  Leq=1e-4 H  R_1=0.01 Ohm  L_1=0.0001 H  R_2=0.01 Ohm  L_2=0.0001 H  averaging_period=0 s  R_m=100 Ohm  parameterization_option=1  H_data=[0, 200, 400, 600, 800, 1000] A/m  B_data=[0, .81, 1.25, 1.42, 1.48, 1.49] T  length_effective=0.2 m  area_effective=2e-4 m^2  L=4e-2 H  L_sat=1e-2 H  current_data=[0, .4, .8, 1.2, 1.6, 2] A  magnetic_flux_data=[0, .161, .25, .284, .295, .299] .* 1e-3 Wb  magnetic_flux_sat=1.6e-04 Wb  dBdH0=0.005 m*T/A  B1=1.49 T  H1=1000 A/m  c=0.1  K=200 A/m  alpha=1e-4  interpolation_option=1  Leq_i0=0 A  L1_i0=0 A  L2_i0=0 A  x0_option=1  i_L0=0 A  phi0=0 Wb  B0=0 T  H0=0 A/m  Leq_g=1e-9 1/Ohm  L1_g=1e-9 1/Ohm  L2_g=1e-9 1/Ohm
      settings: InternalSimscapePortConfiguration="{\"Bottom\":[],\"Left\":[{\"id\":\"p1\",\"label\":\"1+\",\"type\":\"foundation.electrical.electrical\"},{\"id\":\"n1\",\"label\":\"1-\",\"type\":\"foundation.electrical.electrical\"}],\"Right\":[{\"id\":\"p2\",\"label\":\"2+\",\"type\":\"foundation.electrical.electrical\"},{\"id\":\"n2\",\"label\":\"2-\",\"type\":\"foundation.electrical.electrical\"}],\"Top\":[]}"
  PS-Simulink Converter1 : nesl_utility/PS-Simulink Converter  PhysicalDomain=network_engine_domain  SubClassName=ps_output  LeftPortType=input  RightPortType=output  PseudoPeriodic=off  Frequencies=[]  VectorFormat=1-D array  Unit=inherit  AffineConversion=off
  Phase Splitter : ee_lib/Connectors & References/Phase Splitter
  Phase Splitter1 : ee_lib/Connectors & References/Phase Splitter
  Phase Voltage Sensor (Three-Phase)1 : ee_lib/Sensors & Transducers/Phase Voltage Sensor (Three-Phase)
      settings: LogSimulationData=on  InternalSimscapePortConfiguration="{\"Bottom\":[],\"Left\":[{\"id\":\"a1\",\"label\":\"a1\",\"type\":\"foundation.electrical.electrical\"},{\"id\":\"b1\",\"label\":\"b1\",\"type\":\"foundation.electrical.electrical\"},{\"id\":\"c1\",\"label\":\"c1\",\"type\":\"foundation.electrical.electrical\"}],\"Right\":[{\"id\":\"V_output\",\"label\":\"V\",\"type\":\"output\"},{\"id\":\"a2\",\"label\":\"a2\",\"type\":\"foundation.electrical.electrical\"},{\"id\":\"b2\",\"label\":\"b2\",\"type\":\"foundation.electrical.electrical\"},{\"id\":\"c2\",\"label\":\"c2\",\"type\":\"foundation.electrical.electrical\"}],\"Top\":[]}"
  Resistor : fl_lib/Electrical/Electrical Elements/Resistor  R=1 Ohm  i_specify=off  i_priority=None  i=0 A  i_nominal_specify=off  i_nominal_value=1  i_nominal_unit=A  v_specify=off  v_priority=None  v=0 V  v_nominal_specify=off  v_nominal_value=1  v_nominal_unit=V
  Resistor1 : fl_lib/Electrical/Electrical Elements/Resistor  R=1 Ohm  i_specify=off  i_priority=None  i=0 A  i_nominal_specify=off  i_nominal_value=1  i_nominal_unit=A  v_specify=off  v_priority=None  v=0 V  v_nominal_specify=off  v_nominal_value=1  v_nominal_unit=V
  Resistor2 : fl_lib/Electrical/Electrical Elements/Resistor  R=1 Ohm  i_specify=off  i_priority=None  i=0 A  i_nominal_specify=off  i_nominal_value=1  i_nominal_unit=A  v_specify=off  v_priority=None  v=0 V  v_nominal_specify=off  v_nominal_value=1  v_nominal_unit=V
  Sensor dynamics : Subsystem
  ABC1 : PMIOPort  Side=Left
  ABC2 : PMIOPort  Port=2  Side=Right
  Out1 : Outport
  wires:
  PS-Simulink Converter1/1 -> Sensor dynamics/1(V)
  Sensor dynamics/1(I) -> Out1/1
  connections:
  Phase Splitter/LConn1 -- ABC1/RConn1
  ABC2/RConn1 -- Phase Splitter1/LConn1
  Connection Label19/LConn1 -- Phase Voltage Sensor (Three-Phase)1/LConn3
  Connection Label18/LConn1 -- Phase Voltage Sensor (Three-Phase)1/LConn2
  PS-Simulink Converter1/LConn1 -- Phase Voltage Sensor (Three-Phase)1/RConn1
  Connection Label20/LConn1 -- Phase Voltage Sensor (Three-Phase)1/LConn1
  Nonlinear Transformer/RConn1 -- Resistor/LConn1 -- Connection Label12/LConn1
  Nonlinear Transformer/LConn1 -- Phase Splitter/RConn1
  Phase Splitter1/RConn1 -- Nonlinear Transformer/LConn2
  Nonlinear Transformer/RConn2 -- Resistor/RConn1 -- Connection Label1/LConn1
  Nonlinear Transformer1/RConn1 -- Resistor1/LConn1 -- Connection Label3/LConn1
  Nonlinear Transformer1/LConn2 -- Phase Splitter1/RConn2
  Nonlinear Transformer1/LConn1 -- Phase Splitter/RConn2
  Resistor2/LConn1 -- Nonlinear Transformer2/RConn1 -- Connection Label8/LConn1
  Nonlinear Transformer2/LConn1 -- Phase Splitter/RConn3
  Phase Splitter1/RConn3 -- Nonlinear Transformer2/LConn2
  Nonlinear Transformer2/RConn2 -- Resistor2/RConn1 -- Connection Label4/LConn1
  Connection Label2/LConn1 -- Resistor1/RConn1 -- Nonlinear Transformer1/RConn2
  Phase Voltage Sensor (Three-Phase)1/RConn2 -- Phase Voltage Sensor (Three-Phase)1/RConn3 -- Electrical Reference/LConn1 -- Phase Voltage Sensor (Three-Phase)1/RConn4
  Connection Label5/LConn1 -- Grounded Neutral (Three-Phase)1/LConn1
  Connection Label6/LConn1 -- Grounded Neutral (Three-Phase)1/LConn2
  Connection Label7/LConn1 -- Grounded Neutral (Three-Phase)1/LConn3

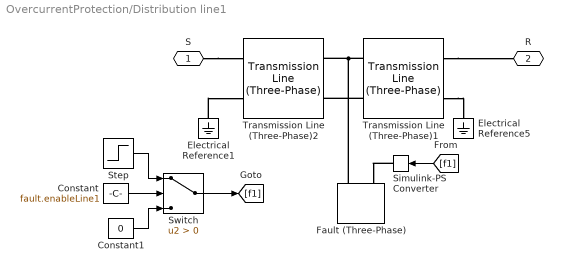
== system OvercurrentProtection/Distribution line1 ==
  Constant : Constant  Value=fault.enableLine1
  Constant1 : Constant  Value=0
  Electrical Reference1 : fl_lib/Electrical/Electrical Elements/Electrical Reference
  Electrical Reference5 : fl_lib/Electrical/Electrical Elements/Electrical Reference
  Fault (Three-Phase) : ee_lib/Utilities/Fault (Three-Phase)  fault_type_option=7  R_pn_fault=1e-6 Ohm  R_ng_fault=1e-6 Ohm  exposemeasurement=ee.enum.exposemeasurement.hidden  enable_external_fault=ee.enum.external_fault.visible  fault_threshold=0.5  fault_condition=1  fault_resettable=1  enable_temporal_fault=0  fault_start_time=0.2 s  fault_duration=0.05 s  G_parasitic=1e-6 1/Ohm
      settings: InternalSimscapePortConfiguration="{\"Bottom\":[],\"Left\":[{\"id\":\"N\",\"label\":\"~\",\"type\":\"foundation.electrical.three_phase\"},{\"id\":\"F\",\"label\":\"F\",\"type\":\"input\"}],\"Right\":[],\"Top\":[]}"
  Simulink-PS Converter : nesl_utility/Simulink-PS Converter  PhysicalDomain=network_engine_domain  SubClassName=ps_input  LeftPortType=input  RightPortType=output  PseudoPeriodic=off  Frequencies=[]  NoiseDistribution=none  NoiseParameters=[]  Unit=1  AffineConversion=off  FilteringAndDerivatives=provide  SimscapeFilterOrder=1  InputFilterTimeConstant=0.001  UdotUserProvided=0
  Step : Step  Time=fault.startTime  SampleTime=0
  Switch : Switch  Criteria=u2 > Threshold  SaturateOnIntegerOverflow=off  InputSameDT=off
  Transmission Line (Three-Phase)1 : ee_lib/Passive/Lines/Transmission Line (Three-Phase)  length=distributionLine1.length-distributionLine1.fault km  freq=60 Hz  R=distributionLine1.resistance Ohm/km  L=distributionLine1.inductance mH/km  M=0 mH/km  Cl=distributionLine1.capacitanceLL uF/km  Cg=distributionLine1.capacitanceLG uF/km  Rm=0 Ohm/km  ModelTwoSections=ee.enum.enable.no  N=1  InterfacePosition=0.5 km  N1sec=1  N2sec=1  Access_ground=ee.enum.enable.no  R_parasitic=1e-4 Ohm  G_parasitic=1e-4 1/Ohm  EnableFault=false  fault_type_option=ee.enum.fault_type_option.ag  R_pn_fault=1e-3 Ohm  R_ng_fault=1e-3 Ohm  unfaulted_G_parasitic=1e-6 1/Ohm
      settings: InternalSimscapePortConfiguration="{\"Bottom\":[],\"Left\":[{\"id\":\"N1\",\"label\":\"~1\",\"type\":\"foundation.electrical.three_phase\"},{\"id\":\"g1\",\"label\":\"g1\",\"type\":\"foundation.electrical.electrical\"}],\"Right\":[{\"id\":\"N2\",\"label\":\"~2\",\"type\":\"foundation.electrical.three_phase\"},{\"id\":\"g2\",\"label\":\"g2\",\"type\":\"foundation.electrical.electrical\"}],\"Top\":[]}"
  Transmission Line (Three-Phase)2 : ee_lib/Passive/Lines/Transmission Line (Three-Phase)  length=distributionLine1.fault km  freq=60 Hz  R=distributionLine1.resistance Ohm/km  L=distributionLine1.inductance mH/km  M=0 mH/km  Cl=distributionLine1.capacitanceLL uF/km  Cg=distributionLine1.capacitanceLG uF/km  Rm=0 Ohm/km  ModelTwoSections=ee.enum.enable.no  N=1  InterfacePosition=0.5 km  N1sec=1  N2sec=1  Access_ground=ee.enum.enable.no  R_parasitic=1e-4 Ohm  G_parasitic=1e-4 1/Ohm  EnableFault=false  fault_type_option=ee.enum.fault_type_option.ag  R_pn_fault=1e-3 Ohm  R_ng_fault=1e-3 Ohm  unfaulted_G_parasitic=1e-6 1/Ohm
      settings: InternalSimscapePortConfiguration="{\"Bottom\":[],\"Left\":[{\"id\":\"N1\",\"label\":\"~1\",\"type\":\"foundation.electrical.three_phase\"},{\"id\":\"g1\",\"label\":\"g1\",\"type\":\"foundation.electrical.electrical\"}],\"Right\":[{\"id\":\"N2\",\"label\":\"~2\",\"type\":\"foundation.electrical.three_phase\"},{\"id\":\"g2\",\"label\":\"g2\",\"type\":\"foundation.electrical.electrical\"}],\"Top\":[]}"
  S : PMIOPort  Side=Left
  R : PMIOPort  Port=2  Side=Right
  wires:
  [f1] -> Simulink-PS Converter/1
  Constant1/1 -> Switch/3
  Step/1 -> Switch/1
  Switch/1 -> [f1]
  Constant/1 -> Switch/2
  connections:
  S/RConn1 -- Transmission Line (Three-Phase)2/LConn1
  Transmission Line (Three-Phase)1/LConn2 -- Transmission Line (Three-Phase)2/RConn2
  Electrical Reference1/LConn1 -- Transmission Line (Three-Phase)2/LConn2
  Transmission Line (Three-Phase)1/RConn2 -- Electrical Reference5/LConn1
  Fault (Three-Phase)/LConn1 -- Transmission Line (Three-Phase)1/LConn1 -- Transmission Line (Three-Phase)2/RConn1
  Transmission Line (Three-Phase)1/RConn1 -- R/RConn1
  Simulink-PS Converter/RConn1 -- Fault (Three-Phase)/LConn2

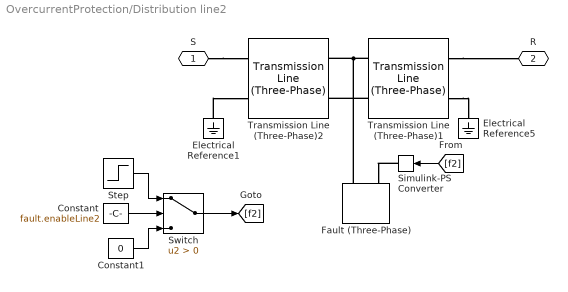
== system OvercurrentProtection/Distribution line2 ==
  Constant : Constant  Value=fault.enableLine2
  Constant1 : Constant  Value=0
  Electrical Reference1 : fl_lib/Electrical/Electrical Elements/Electrical Reference
  Electrical Reference5 : fl_lib/Electrical/Electrical Elements/Electrical Reference
  Fault (Three-Phase) : ee_lib/Utilities/Fault (Three-Phase)  fault_type_option=1  R_pn_fault=1e-6 Ohm  R_ng_fault=1e-6 Ohm  exposemeasurement=ee.enum.exposemeasurement.hidden  enable_external_fault=ee.enum.external_fault.visible  fault_threshold=0.5  fault_condition=1  fault_resettable=1  enable_temporal_fault=0  fault_start_time=0.2 s  fault_duration=0.05 s  G_parasitic=1e-6 1/Ohm
      settings: InternalSimscapePortConfiguration="{\"Bottom\":[],\"Left\":[{\"id\":\"N\",\"label\":\"~\",\"type\":\"foundation.electrical.three_phase\"},{\"id\":\"F\",\"label\":\"F\",\"type\":\"input\"}],\"Right\":[],\"Top\":[]}"
  Simulink-PS Converter : nesl_utility/Simulink-PS Converter  PhysicalDomain=network_engine_domain  SubClassName=ps_input  LeftPortType=input  RightPortType=output  PseudoPeriodic=off  Frequencies=[]  NoiseDistribution=none  NoiseParameters=[]  Unit=1  AffineConversion=off  FilteringAndDerivatives=provide  SimscapeFilterOrder=1  InputFilterTimeConstant=0.001  UdotUserProvided=0
  Step : Step  Time=fault.startTime  SampleTime=0
  Switch : Switch  Criteria=u2 > Threshold  SaturateOnIntegerOverflow=off  InputSameDT=off
  Transmission Line (Three-Phase)1 : ee_lib/Passive/Lines/Transmission Line (Three-Phase)  length=distributionLine2.length-distributionLine2.fault km  freq=60 Hz  R=distributionLine2.resistance Ohm/km  L=distributionLine2.inductance mH/km  M=0 mH/km  Cl=distributionLine2.capacitanceLL uF/km  Cg=distributionLine2.capacitanceLG uF/km  Rm=0 Ohm/km  ModelTwoSections=ee.enum.enable.no  N=1  InterfacePosition=0.5 km  N1sec=1  N2sec=1  Access_ground=ee.enum.enable.no  R_parasitic=1e-6 Ohm  G_parasitic=1e-6 1/Ohm  EnableFault=false  fault_type_option=ee.enum.fault_type_option.ag  R_pn_fault=1e-3 Ohm  R_ng_fault=1e-3 Ohm  unfaulted_G_parasitic=1e-6 1/Ohm
      settings: InternalSimscapePortConfiguration="{\"Bottom\":[],\"Left\":[{\"id\":\"N1\",\"label\":\"~1\",\"type\":\"foundation.electrical.three_phase\"},{\"id\":\"g1\",\"label\":\"g1\",\"type\":\"foundation.electrical.electrical\"}],\"Right\":[{\"id\":\"N2\",\"label\":\"~2\",\"type\":\"foundation.electrical.three_phase\"},{\"id\":\"g2\",\"label\":\"g2\",\"type\":\"foundation.electrical.electrical\"}],\"Top\":[]}"
  Transmission Line (Three-Phase)2 : ee_lib/Passive/Lines/Transmission Line (Three-Phase)  length=distributionLine2.fault km  freq=60 Hz  R=distributionLine2.resistance Ohm/km  L=distributionLine2.inductance mH/km  M=0 mH/km  Cl=distributionLine2.capacitanceLL uF/km  Cg=distributionLine2.capacitanceLG uF/km  Rm=0 Ohm/km  ModelTwoSections=ee.enum.enable.no  N=1  InterfacePosition=0.5 km  N1sec=1  N2sec=1  Access_ground=ee.enum.enable.no  R_parasitic=1e-4 Ohm  G_parasitic=1e-4 1/Ohm  EnableFault=false  fault_type_option=ee.enum.fault_type_option.ag  R_pn_fault=1e-3 Ohm  R_ng_fault=1e-3 Ohm  unfaulted_G_parasitic=1e-6 1/Ohm
      settings: InternalSimscapePortConfiguration="{\"Bottom\":[],\"Left\":[{\"id\":\"N1\",\"label\":\"~1\",\"type\":\"foundation.electrical.three_phase\"},{\"id\":\"g1\",\"label\":\"g1\",\"type\":\"foundation.electrical.electrical\"}],\"Right\":[{\"id\":\"N2\",\"label\":\"~2\",\"type\":\"foundation.electrical.three_phase\"},{\"id\":\"g2\",\"label\":\"g2\",\"type\":\"foundation.electrical.electrical\"}],\"Top\":[]}"
  S : PMIOPort  Side=Left
  R : PMIOPort  Port=2  Side=Right
  wires:
  [f2] -> Simulink-PS Converter/1
  Constant/1 -> Switch/2
  Constant1/1 -> Switch/3
  Step/1 -> Switch/1
  Switch/1 -> [f2]
  connections:
  S/RConn1 -- Transmission Line (Three-Phase)2/LConn1
  Transmission Line (Three-Phase)1/LConn2 -- Transmission Line (Three-Phase)2/RConn2
  Electrical Reference1/LConn1 -- Transmission Line (Three-Phase)2/LConn2
  Transmission Line (Three-Phase)1/RConn2 -- Electrical Reference5/LConn1
  Fault (Three-Phase)/LConn1 -- Transmission Line (Three-Phase)2/RConn1 -- Transmission Line (Three-Phase)1/LConn1
  Transmission Line (Three-Phase)1/RConn1 -- R/RConn1
  Simulink-PS Converter/RConn1 -- Fault (Three-Phase)/LConn2
